simulink model "WT_gearlife"  (R2020a)
settings: Solver=VariableStepAuto  StartTime=0.0  StopTime=10  MaxStep=.01  RelTol=1e-3
undefined symbols (not defined in the file): b1, b2, b3, CD2, CD3, cosPhi, ds, E, m2, m3, rs, T1, T2, T3, TR1, TR2, TR3, y2, y3, ym, yp
settings Model: Creator=Jayan Joshua  LastModifiedBy=Jayan Joshua

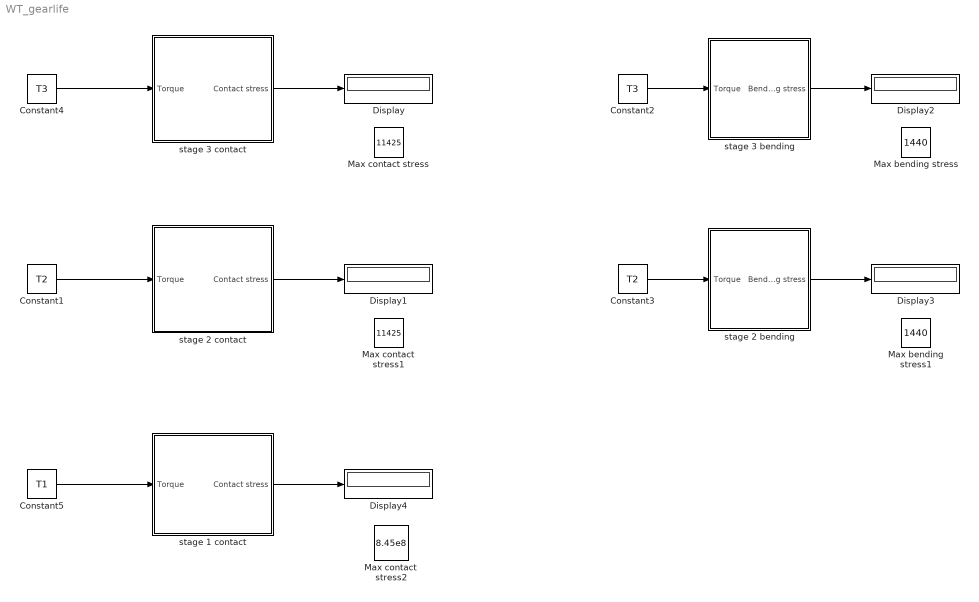
== system WT_gearlife ==
  Constant1 : Constant  Value=T2
  Constant2 : Constant  Value=T3
  Constant3 : Constant  Value=T2
  Constant4 : Constant  Value=T3
  Constant5 : Constant  Value=T1
  Display{,1..4} (5 alike) : Display
  Max bending stress : Constant  Value=1440
  Max bending stress1 : Constant  Value=1440
  Max contact stress : Constant  Value=11425
  Max contact stress1 : Constant  Value=11425
  Max contact stress2 : Constant  Value=8.45e8
  stage 1 contact : Subsystem
  stage 2 bending : Subsystem
  stage 2 contact : Subsystem
  stage 3 bending : Subsystem
  stage 3 contact : Subsystem
  wires:
  stage 3 contact/1(Contact stress) -> Display/1
  Constant4/1 -> stage 3 contact/1(Torque)
  Constant1/1 -> stage 2 contact/1(Torque)
  stage 2 contact/1(Contact stress) -> Display1/1
  Constant2/1 -> stage 3 bending/1(Torque)
  stage 3 bending/1(Bending stress) -> Display2/1
  stage 2 bending/1(Bending stress) -> Display3/1
  Constant3/1 -> stage 2 bending/1(Torque)
  Constant5/1 -> stage 1 contact/1(Torque)
  stage 1 contact/1(Contact stress) -> Display4/1

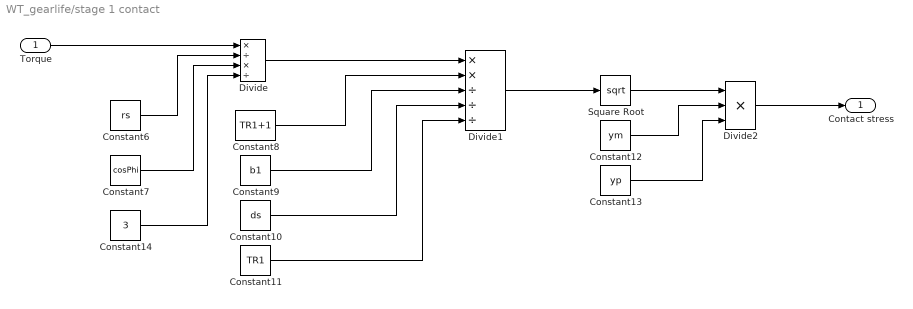
== system WT_gearlife/stage 1 contact ==
  Torque : Inport
  Constant10 : Constant  Value=ds
  Constant11 : Constant  Value=TR1
  Constant12 : Constant  Value=ym
  Constant13 : Constant  Value=yp
  Constant14 : Constant  Value=3
  Constant6 : Constant  Value=rs
  Constant7 : Constant  Value=cosPhi
  Constant8 : Constant  Value=TR1+1
  Constant9 : Constant  Value=b1
  Divide : Product  Inputs=*/*/
  Divide1 : Product  Inputs=**///
  Divide2 : Product  Inputs=***
  Square Root : Sqrt  SaturateOnIntegerOverflow=on
  Contact stress : Outport
  wires:
  Square Root/1 -> Divide2/1
  Constant6/1 -> Divide/2
  Constant10/1 -> Divide1/4
  Constant13/1 -> Divide2/3
  Constant7/1 -> Divide/3
  Constant8/1 -> Divide1/2
  Constant11/1 -> Divide1/5
  Constant14/1 -> Divide/4
  Constant9/1 -> Divide1/3
  Divide/1 -> Divide1/1
  Divide1/1 -> Square Root/1
  Constant12/1 -> Divide2/2
  Divide2/1 -> Contact stress/1
  Torque/1 -> Divide/1

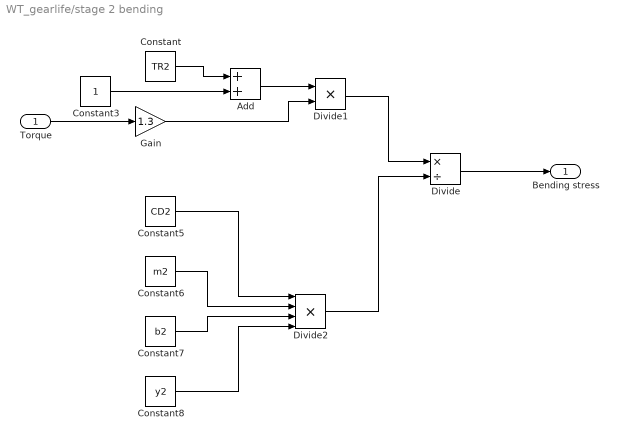
== system WT_gearlife/stage 2 bending ==
  Torque : Inport
  Add : Sum
  Constant : Constant  Value=TR2
  Constant3 : Constant
  Constant5 : Constant  Value=CD2
  Constant6 : Constant  Value=m2
  Constant7 : Constant  Value=b2
  Constant8 : Constant  Value=y2
  Divide : Product  Inputs=*/
  Divide1 : Product  Inputs=**
  Divide2 : Product  Inputs=****
  Gain : Gain  Gain=1.3
  Bending stress : Outport
  wires:
  Torque/1 -> Gain/1
  Divide/1 -> Bending stress/1
  Constant5/1 -> Divide2/1
  Divide2/1 -> Divide/2
  Add/1 -> Divide1/1
  Constant8/1 -> Divide2/4
  Constant/1 -> Add/1
  Gain/1 -> Divide1/2
  Divide1/1 -> Divide/1
  Constant7/1 -> Divide2/3
  Constant6/1 -> Divide2/2
  Constant3/1 -> Add/2

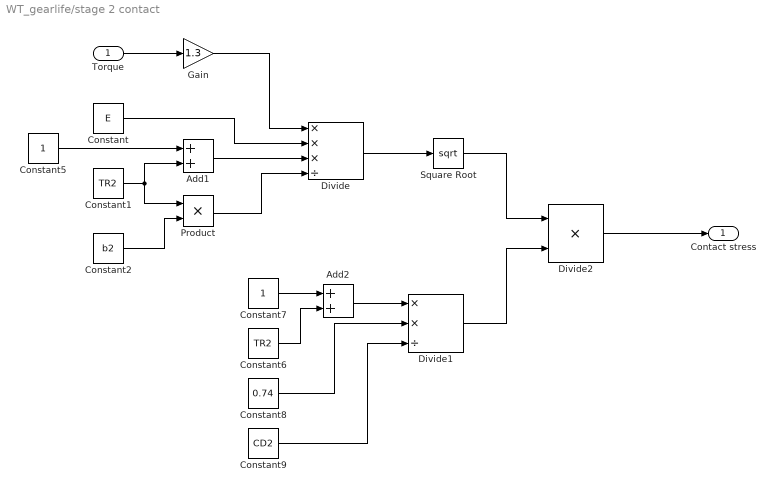
== system WT_gearlife/stage 2 contact ==
  Torque : Inport
  Add1 : Sum
  Add2 : Sum
  Constant : Constant  Value=E
  Constant1 : Constant  Value=TR2
  Constant2 : Constant  Value=b2
  Constant5 : Constant
  Constant6 : Constant  Value=TR2
  Constant7 : Constant
  Constant8 : Constant  Value=0.74
  Constant9 : Constant  Value=CD2
  Divide : Product  Inputs=***/
  Divide1 : Product  Inputs=**/
  Divide2 : Product  Inputs=**
  Gain : Gain  Gain=1.3
  Product : Product
  Square Root : Sqrt  SaturateOnIntegerOverflow=on
  Contact stress : Outport
  wires:
  Torque/1 -> Gain/1
  Add2/1 -> Divide1/1
  Constant6/1 -> Add2/2
  Divide/1 -> Square Root/1
  Gain/1 -> Divide/1
  Constant/1 -> Divide/2
  Constant1/1 -> Add1/2, Product/1
  Divide1/1 -> Divide2/2
  Add1/1 -> Divide/3
  Constant2/1 -> Product/2
  Divide2/1 -> Contact stress/1
  Constant5/1 -> Add1/1
  Constant8/1 -> Divide1/2
  Constant7/1 -> Add2/1
  Product/1 -> Divide/4
  Square Root/1 -> Divide2/1
  Constant9/1 -> Divide1/3

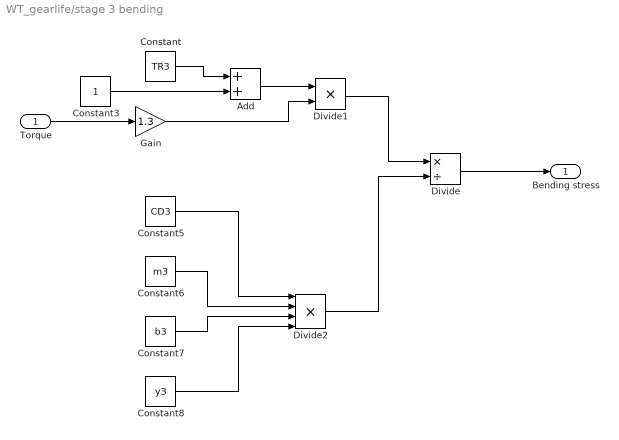
== system WT_gearlife/stage 3 bending ==
  Torque : Inport
  Add : Sum
  Constant : Constant  Value=TR3
  Constant3 : Constant
  Constant5 : Constant  Value=CD3
  Constant6 : Constant  Value=m3
  Constant7 : Constant  Value=b3
  Constant8 : Constant  Value=y3
  Divide : Product  Inputs=*/
  Divide1 : Product  Inputs=**
  Divide2 : Product  Inputs=****
  Gain : Gain  Gain=1.3
  Bending stress : Outport
  wires:
  Constant3/1 -> Add/2
  Constant6/1 -> Divide2/2
  Constant7/1 -> Divide2/3
  Divide1/1 -> Divide/1
  Gain/1 -> Divide1/2
  Constant/1 -> Add/1
  Constant8/1 -> Divide2/4
  Add/1 -> Divide1/1
  Divide2/1 -> Divide/2
  Constant5/1 -> Divide2/1
  Divide/1 -> Bending stress/1
  Torque/1 -> Gain/1

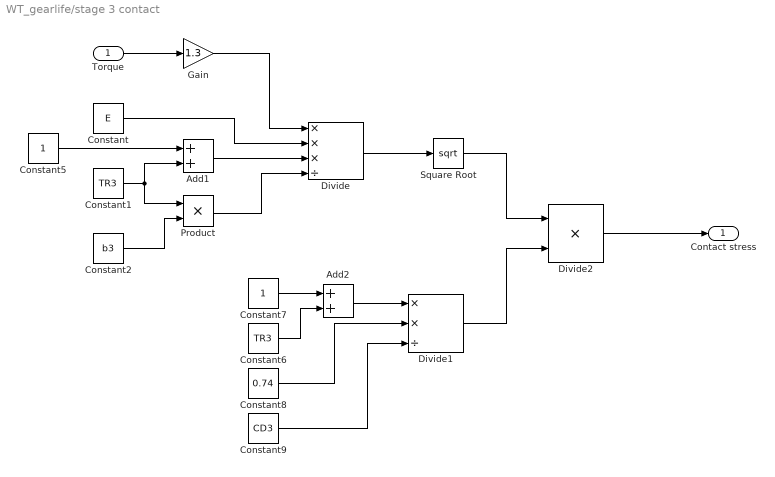
== system WT_gearlife/stage 3 contact ==
  Torque : Inport
  Add1 : Sum
  Add2 : Sum
  Constant : Constant  Value=E
  Constant1 : Constant  Value=TR3
  Constant2 : Constant  Value=b3
  Constant5 : Constant
  Constant6 : Constant  Value=TR3
  Constant7 : Constant
  Constant8 : Constant  Value=0.74
  Constant9 : Constant  Value=CD3
  Divide : Product  Inputs=***/
  Divide1 : Product  Inputs=**/
  Divide2 : Product  Inputs=**
  Gain : Gain  Gain=1.3
  Product : Product
  Square Root : Sqrt  SaturateOnIntegerOverflow=on
  Contact stress : Outport
  wires:
  Constant9/1 -> Divide1/3
  Square Root/1 -> Divide2/1
  Product/1 -> Divide/4
  Constant7/1 -> Add2/1
  Constant8/1 -> Divide1/2
  Constant5/1 -> Add1/1
  Divide2/1 -> Contact stress/1
  Constant2/1 -> Product/2
  Add1/1 -> Divide/3
  Divide1/1 -> Divide2/2
  Constant1/1 -> Product/1, Add1/2
  Constant/1 -> Divide/2
  Gain/1 -> Divide/1
  Divide/1 -> Square Root/1
  Constant6/1 -> Add2/2
  Add2/1 -> Divide1/1
  Torque/1 -> Gain/1
